simulink model "SplROMInt"  (Simulink 4.00)
settings: Solver=FixedStepDiscrete  StartTime=0.0  StopTime=1024  RelTol=1e-3
libraries: bus_alteradspbuilder x56, store_alteradspbuilder x51, arithm_alteradspbuilder x13
Description:
  | 10 разрядный сплайн-интерполятор
  | Увеличивает частоту дискретизации в кратное двум
  | число раз
  | Использована интерполяция кубическим эрмитовым
  | сплайном
settings Model: Creator="Igor Shelevitsky  sheleviv@mail.ru"  LastModifiedBy=igors

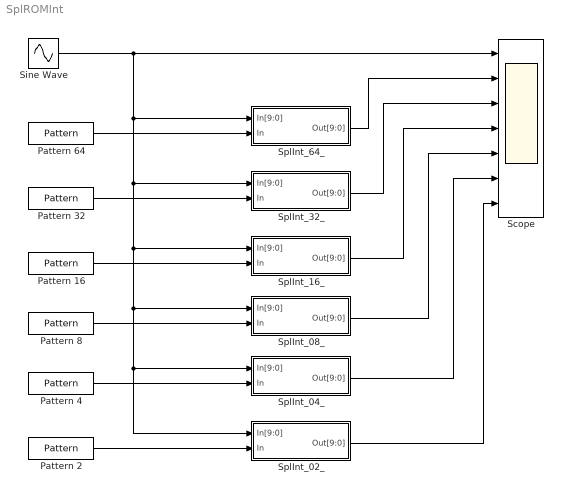
== system SplROMInt ==
  Pattern {2,4,8,16,32,64} (6 alike) : store_alteradspbuilder/Pattern  Priority=28  clken=off  ntsamp=1
  Scope : Scope  NumInputPorts=7
      settings: TimeRange=1024  YMin=-512~-512~-512~-512~-512~-512~-512  YMax=512~512~512~512~512~512~512  SaveToWorkspace=off  SaveName=ScopeData  LimitDataPoints=on  MaxDataPoints=5000
  Sine Wave : Sin  SineType=Time-based  Amplitude=511  Bias=0  Frequency=0.02  Phase=0  Samples=10  SampleTime=1  Offset=0
  SplInt_02_ : Subsystem  AncestorBlock=ALTELINK/AltLab/HDL SubSystem
      settings: RTWFcnNameOpts=Auto  RTWFileNameOpts=Auto
      mask Type: SubSystem AlteraBlockSet
  SplInt_04_ : Subsystem  AncestorBlock=ALTELINK/AltLab/HDL SubSystem
      settings: RTWFcnNameOpts=Auto  RTWFileNameOpts=Auto
      mask Type: SubSystem AlteraBlockSet
  SplInt_08_ : Subsystem  AncestorBlock=ALTELINK/AltLab/HDL SubSystem
      settings: RTWFcnNameOpts=Auto  RTWFileNameOpts=Auto
      mask Type: SubSystem AlteraBlockSet
  SplInt_16_ : Subsystem  AncestorBlock=ALTELINK/AltLab/HDL SubSystem
      settings: RTWFcnNameOpts=Auto  RTWFileNameOpts=Auto
      mask Type: SubSystem AlteraBlockSet
  SplInt_32_ : Subsystem  AncestorBlock=ALTELINK/AltLab/HDL SubSystem
      settings: RTWFcnNameOpts=Auto  RTWFileNameOpts=Auto
      mask Type: SubSystem AlteraBlockSet
  "SplInt_64_ " : Subsystem  AncestorBlock=ALTELINK/AltLab/HDL SubSystem
      settings: RTWFcnNameOpts=Auto  RTWFileNameOpts=Auto
      mask Type: SubSystem AlteraBlockSet
  wires:
  Sine Wave/1 -> "SplInt_64_ "/1(In[9:0]), SplInt_04_/1(In[9:0]), SplInt_02_/1(In[9:0]), SplInt_08_/1(In[9:0]), SplInt_16_/1(In[9:0]), SplInt_32_/1(In[9:0]), Scope/1
  "SplInt_64_ "/1(Out[9:0]) -> Scope/2
  SplInt_32_/1(Out[9:0]) -> Scope/3
  SplInt_16_/1(Out[9:0]) -> Scope/4
  SplInt_08_/1(Out[9:0]) -> Scope/5
  SplInt_04_/1(Out[9:0]) -> Scope/6
  SplInt_02_/1(Out[9:0]) -> Scope/7
  Pattern 64/1 -> "SplInt_64_ "/2(In)
  Pattern 32/1 -> SplInt_32_/2(In)
  Pattern 16/1 -> SplInt_16_/2(In)
  Pattern 8/1 -> SplInt_08_/2(In)
  Pattern 4/1 -> SplInt_04_/2(In)
  Pattern 2/1 -> SplInt_02_/2(In)

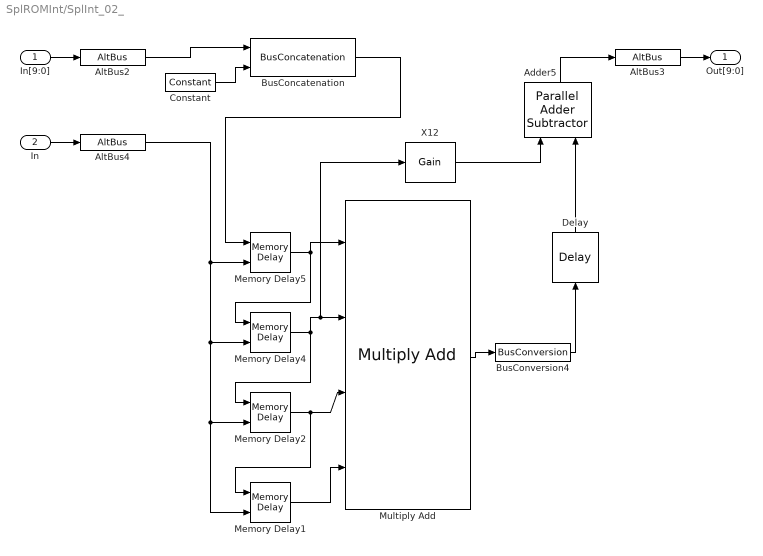
== system SplROMInt/SplInt_02_ ==
  In[9:0] : Inport  Port=1  LatchInput=off
  In : Inport  Port=2  LatchInput=off
  Adder5 : arithm_alteradspbuilder/Parallel  Adder Subtractor  Orientation=up  Inputs=2  direction=++  pipeline=off  clken=off  MaskValue=1
  AltBus2 : bus_alteradspbuilder/AltBus  Description=Sign Binary Fractionnal  sgn=Signed Integer  nodetype=Input Port  bwl=10  bwr=8  sat=off  rnd=off  bp=off  mask_cst=0  LocPin=any  cst=0  modulename=AltBus2  nSgCpl=0
  AltBus3 : bus_alteradspbuilder/AltBus  Description=Sign Binary Fractionnal  sgn=Signed Integer  nodetype=Output Port  bwl=10  bwr=8  sat=off  rnd=off  bp=off  mask_cst=0  LocPin=any  cst=0  modulename=AltBus3  nSgCpl=0
  AltBus4 : bus_alteradspbuilder/AltBus  Description=Sign Binary Fractionnal  sgn=Single Bit  nodetype=Input Port  bwl=1  bwr=0  sat=off  rnd=off  bp=off  mask_cst=0  LocPin=any  cst=0  modulename=AltBus4  nSgCpl=0
  BusConcatenation : bus_alteradspbuilder/BusConcatenation  bwl=10  bwr=4  blean=on
  BusConversion4 : bus_alteradspbuilder/BusConversion  Inputs=Signed Integer  bwl=26  bwr=8  Outputs=Signed Integer  obwl=10  obwr=0  msb=25  lsb=16  rnd=off  sat=off
  Constant : bus_alteradspbuilder/Constant  Description=Sign Binary Fractionnal  sgn=Unsigned Integer  nodetype=Constant  bwl=4  bwr=8  sat=off  rnd=off  bp=off  mask_cst=0  ncstsamp=1  cst=0  modulename=Constant  nSgCpl=0
  Delay : store_alteradspbuilder/Delay  Orientation=up  depth=1  clken=off  MaskValue=1
  Memory Delay{1..2,4..5} (4 alike) : store_alteradspbuilder/Memory Delay  bwaddr=1  depth=1  cst=off  clken=on  eab=on  vDepthAltr=1
  Multiply Add : arithm_alteradspbuilder/Multiply Add  depth=4  BusType=Signed Integer  bwl=14  bwr=0  direction=Add Add  pipeline=No Register  clken=off  eab=off  cst=on  Constantvalues=[-256 2304 2304 -256]  gain=[-256.000000,2304.000000,2304.000000,-256.000000]
  X12 : arithm_alteradspbuilder/Gain  vgain=4096  BusType=Signed Integer  bwl=14  bwr=0  pipeline=0  lpm=off  clken=off  gain=4096  MaskValue=1
  Out[9:0] : Outport  Port=1
  wires:
  AltBus3/1 -> Out[9:0]/1
  In[9:0]/1 -> AltBus2/1
  Multiply Add/1 -> BusConversion4/1
  Memory Delay5/1 -> Memory Delay4/1, Multiply Add/1
  Memory Delay4/1 -> Memory Delay2/1, Multiply Add/2, X12/1
  Memory Delay2/1 -> Memory Delay1/1, Multiply Add/3
  Memory Delay1/1 -> Multiply Add/4
  In/1 -> AltBus4/1
  BusConversion4/1 -> Delay/1
  AltBus4/1 -> Memory Delay5/2, Memory Delay4/2, Memory Delay1/2, Memory Delay2/2
  Constant/1 -> BusConcatenation/2
  AltBus2/1 -> BusConcatenation/1
  BusConcatenation/1 -> Memory Delay5/1
  Adder5/1 -> AltBus3/1
  Delay/1 -> Adder5/2
  X12/1 -> Adder5/1

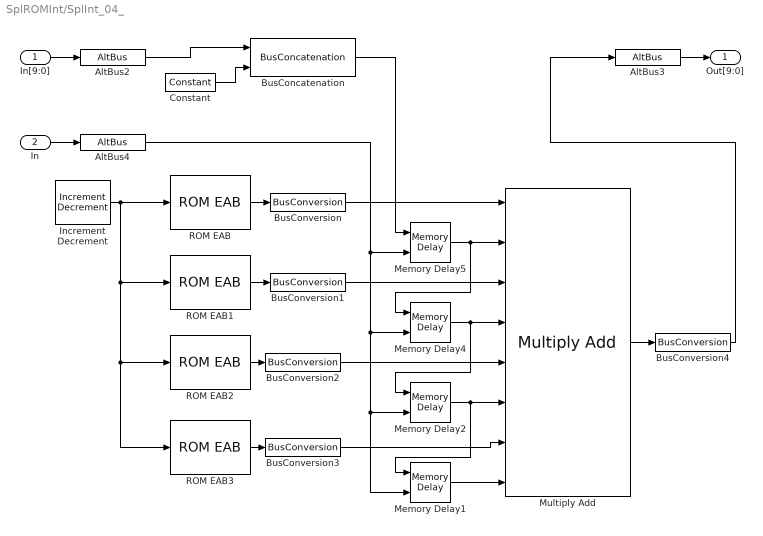
== system SplROMInt/SplInt_04_ ==
  In[9:0] : Inport  Port=1  LatchInput=off
  In : Inport  Port=2  LatchInput=off
  AltBus2 : bus_alteradspbuilder/AltBus  Description=Sign Binary Fractionnal  sgn=Signed Integer  nodetype=Input Port  bwl=10  bwr=8  sat=off  rnd=off  bp=off  mask_cst=0  LocPin=any  cst=0  modulename=AltBus2  nSgCpl=0
  AltBus3 : bus_alteradspbuilder/AltBus  Description=Sign Binary Fractionnal  sgn=Signed Integer  nodetype=Output Port  bwl=10  bwr=8  sat=off  rnd=off  bp=off  mask_cst=0  LocPin=any  cst=0  modulename=AltBus3  nSgCpl=0
  AltBus4 : bus_alteradspbuilder/AltBus  Description=Sign Binary Fractionnal  sgn=Single Bit  nodetype=Input Port  bwl=1  bwr=0  sat=off  rnd=off  bp=off  mask_cst=0  LocPin=any  cst=0  modulename=AltBus4  nSgCpl=0
  BusConcatenation : bus_alteradspbuilder/BusConcatenation  bwl=10  bwr=4  blean=on
  BusConversion{,1..3} (4 alike) : bus_alteradspbuilder/BusConversion  Inputs=Signed Integer  bwl=16  bwr=8  Outputs=Signed Integer  obwl=14  obwr=0  msb=13  lsb=0  rnd=off  sat=off
  BusConversion4 : bus_alteradspbuilder/BusConversion  Inputs=Signed Integer  bwl=26  bwr=8  Outputs=Signed Integer  obwl=10  obwr=0  msb=25  lsb=16  rnd=off  sat=off
  Constant : bus_alteradspbuilder/Constant  Description=Sign Binary Fractionnal  sgn=Unsigned Integer  nodetype=Constant  bwl=4  bwr=8  sat=off  rnd=off  bp=off  mask_cst=0  ncstsamp=1  cst=0  modulename=Constant  nSgCpl=0
  Increment Decrement : arithm_alteradspbuilder/Increment Decrement  BusType=Unsigned Integer  bwl=2  bwr=4  direction=Increment  cst=0  clken=off  ntsamp=1  MaskValue=1
  Memory Delay{1..2,4..5} (4 alike) : store_alteradspbuilder/Memory Delay  bwaddr=1  depth=1  cst=off  clken=on  eab=on  vDepthAltr=1
  Multiply Add : arithm_alteradspbuilder/Multiply Add  depth=4  BusType=Signed Integer  bwl=14  bwr=0  direction=Add Add  pipeline=No Register  clken=off  eab=off  cst=off  Constantvalues=[1 1 1 1]  gain=[1.000000,1.000000,1.000000,1.000000]
  ROM EAB : store_alteradspbuilder/ROM EAB  BusType=Signed Integer  bwl=16  bwr=0  bwaddr=2  Inputs=spl00404.hex  MaskValue=1
  ROM EAB1 : store_alteradspbuilder/ROM EAB  BusType=Signed Integer  bwl=16  bwr=0  bwaddr=2  Inputs=spl00403.hex  MaskValue=1
  ROM EAB2 : store_alteradspbuilder/ROM EAB  BusType=Signed Integer  bwl=16  bwr=0  bwaddr=2  Inputs=spl00402.hex  MaskValue=1
  ROM EAB3 : store_alteradspbuilder/ROM EAB  BusType=Signed Integer  bwl=16  bwr=0  bwaddr=2  Inputs=spl00401.hex  MaskValue=1
  Out[9:0] : Outport  Port=1
  wires:
  AltBus3/1 -> Out[9:0]/1
  In[9:0]/1 -> AltBus2/1
  Increment Decrement/1 -> ROM EAB/1, ROM EAB1/1, ROM EAB2/1, ROM EAB3/1
  ROM EAB/1 -> BusConversion/1
  ROM EAB1/1 -> BusConversion1/1
  ROM EAB2/1 -> BusConversion2/1
  ROM EAB3/1 -> BusConversion3/1
  BusConversion/1 -> Multiply Add/1
  BusConversion1/1 -> Multiply Add/3
  BusConversion2/1 -> Multiply Add/5
  BusConversion3/1 -> Multiply Add/7
  Multiply Add/1 -> BusConversion4/1
  Memory Delay5/1 -> Multiply Add/2, Memory Delay4/1
  Memory Delay4/1 -> Multiply Add/4, Memory Delay2/1
  Memory Delay2/1 -> Multiply Add/6, Memory Delay1/1
  Memory Delay1/1 -> Multiply Add/8
  In/1 -> AltBus4/1
  BusConversion4/1 -> AltBus3/1
  AltBus4/1 -> Memory Delay5/2, Memory Delay4/2, Memory Delay1/2, Memory Delay2/2
  Constant/1 -> BusConcatenation/2
  AltBus2/1 -> BusConcatenation/1
  BusConcatenation/1 -> Memory Delay5/1

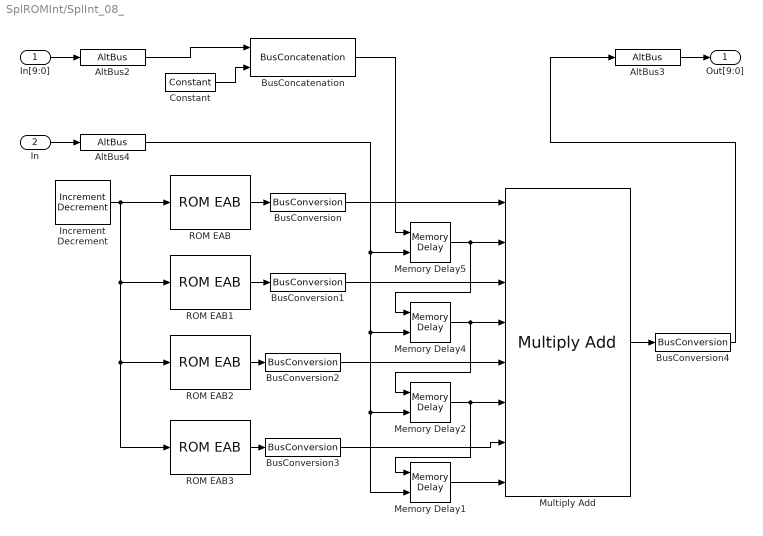
== system SplROMInt/SplInt_08_ ==
  In[9:0] : Inport  Port=1  LatchInput=off
  In : Inport  Port=2  LatchInput=off
  AltBus2 : bus_alteradspbuilder/AltBus  Description=Sign Binary Fractionnal  sgn=Signed Integer  nodetype=Input Port  bwl=10  bwr=8  sat=off  rnd=off  bp=off  mask_cst=0  LocPin=any  cst=0  modulename=AltBus2  nSgCpl=0
  AltBus3 : bus_alteradspbuilder/AltBus  Description=Sign Binary Fractionnal  sgn=Signed Integer  nodetype=Output Port  bwl=10  bwr=8  sat=off  rnd=off  bp=off  mask_cst=0  LocPin=any  cst=0  modulename=AltBus3  nSgCpl=0
  AltBus4 : bus_alteradspbuilder/AltBus  Description=Sign Binary Fractionnal  sgn=Single Bit  nodetype=Input Port  bwl=1  bwr=0  sat=off  rnd=off  bp=off  mask_cst=0  LocPin=any  cst=0  modulename=AltBus4  nSgCpl=0
  BusConcatenation : bus_alteradspbuilder/BusConcatenation  bwl=10  bwr=4  blean=on
  BusConversion{,1..3} (4 alike) : bus_alteradspbuilder/BusConversion  Inputs=Signed Integer  bwl=16  bwr=8  Outputs=Signed Integer  obwl=14  obwr=0  msb=13  lsb=0  rnd=off  sat=off
  BusConversion4 : bus_alteradspbuilder/BusConversion  Inputs=Signed Integer  bwl=26  bwr=8  Outputs=Signed Integer  obwl=10  obwr=0  msb=25  lsb=16  rnd=off  sat=off
  Constant : bus_alteradspbuilder/Constant  Description=Sign Binary Fractionnal  sgn=Unsigned Integer  nodetype=Constant  bwl=4  bwr=8  sat=off  rnd=off  bp=off  mask_cst=0  ncstsamp=1  cst=0  modulename=Constant  nSgCpl=0
  Increment Decrement : arithm_alteradspbuilder/Increment Decrement  BusType=Unsigned Integer  bwl=3  bwr=4  direction=Increment  cst=0  clken=off  ntsamp=1  MaskValue=1
  Memory Delay{1..2,4..5} (4 alike) : store_alteradspbuilder/Memory Delay  bwaddr=1  depth=1  cst=off  clken=on  eab=on  vDepthAltr=1
  Multiply Add : arithm_alteradspbuilder/Multiply Add  depth=4  BusType=Signed Integer  bwl=14  bwr=0  direction=Add Add  pipeline=No Register  clken=off  eab=off  cst=off  Constantvalues=[1 1 1 1]  gain=[1.000000,1.000000,1.000000,1.000000]
  ROM EAB : store_alteradspbuilder/ROM EAB  BusType=Signed Integer  bwl=16  bwr=0  bwaddr=3  Inputs=spl00804.hex  MaskValue=1
  ROM EAB1 : store_alteradspbuilder/ROM EAB  BusType=Signed Integer  bwl=16  bwr=0  bwaddr=3  Inputs=spl00803.hex  MaskValue=1
  ROM EAB2 : store_alteradspbuilder/ROM EAB  BusType=Signed Integer  bwl=16  bwr=0  bwaddr=3  Inputs=spl00802.hex  MaskValue=1
  ROM EAB3 : store_alteradspbuilder/ROM EAB  BusType=Signed Integer  bwl=16  bwr=0  bwaddr=3  Inputs=spl00801.hex  MaskValue=1
  Out[9:0] : Outport  Port=1
  wires:
  AltBus3/1 -> Out[9:0]/1
  In[9:0]/1 -> AltBus2/1
  Increment Decrement/1 -> ROM EAB/1, ROM EAB1/1, ROM EAB2/1, ROM EAB3/1
  ROM EAB/1 -> BusConversion/1
  ROM EAB1/1 -> BusConversion1/1
  ROM EAB2/1 -> BusConversion2/1
  ROM EAB3/1 -> BusConversion3/1
  BusConversion/1 -> Multiply Add/1
  BusConversion1/1 -> Multiply Add/3
  BusConversion2/1 -> Multiply Add/5
  BusConversion3/1 -> Multiply Add/7
  Multiply Add/1 -> BusConversion4/1
  Memory Delay5/1 -> Multiply Add/2, Memory Delay4/1
  Memory Delay4/1 -> Multiply Add/4, Memory Delay2/1
  Memory Delay2/1 -> Multiply Add/6, Memory Delay1/1
  Memory Delay1/1 -> Multiply Add/8
  In/1 -> AltBus4/1
  BusConversion4/1 -> AltBus3/1
  AltBus4/1 -> Memory Delay5/2, Memory Delay4/2, Memory Delay1/2, Memory Delay2/2
  Constant/1 -> BusConcatenation/2
  AltBus2/1 -> BusConcatenation/1
  BusConcatenation/1 -> Memory Delay5/1

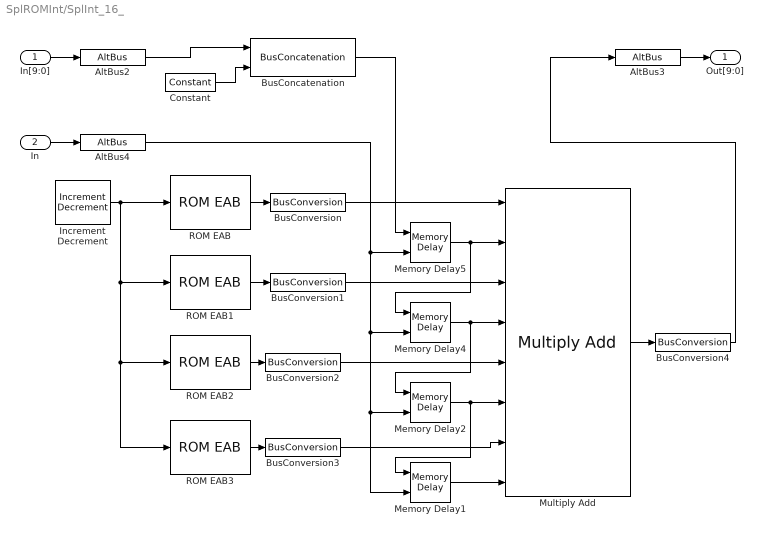
== system SplROMInt/SplInt_16_ ==
  In[9:0] : Inport  Port=1  LatchInput=off
  In : Inport  Port=2  LatchInput=off
  AltBus2 : bus_alteradspbuilder/AltBus  Description=Sign Binary Fractionnal  sgn=Signed Integer  nodetype=Input Port  bwl=10  bwr=8  sat=off  rnd=off  bp=off  mask_cst=0  LocPin=any  cst=0  modulename=AltBus2  nSgCpl=0
  AltBus3 : bus_alteradspbuilder/AltBus  Description=Sign Binary Fractionnal  sgn=Signed Integer  nodetype=Output Port  bwl=10  bwr=8  sat=off  rnd=off  bp=off  mask_cst=0  LocPin=any  cst=0  modulename=AltBus3  nSgCpl=0
  AltBus4 : bus_alteradspbuilder/AltBus  Description=Sign Binary Fractionnal  sgn=Single Bit  nodetype=Input Port  bwl=1  bwr=0  sat=off  rnd=off  bp=off  mask_cst=0  LocPin=any  cst=0  modulename=AltBus4  nSgCpl=0
  BusConcatenation : bus_alteradspbuilder/BusConcatenation  bwl=10  bwr=4  blean=on
  BusConversion{,1..3} (4 alike) : bus_alteradspbuilder/BusConversion  Inputs=Signed Integer  bwl=16  bwr=8  Outputs=Signed Integer  obwl=14  obwr=0  msb=13  lsb=0  rnd=off  sat=off
  BusConversion4 : bus_alteradspbuilder/BusConversion  Inputs=Signed Integer  bwl=26  bwr=8  Outputs=Signed Integer  obwl=10  obwr=0  msb=25  lsb=16  rnd=off  sat=off
  Constant : bus_alteradspbuilder/Constant  Description=Sign Binary Fractionnal  sgn=Unsigned Integer  nodetype=Constant  bwl=4  bwr=8  sat=off  rnd=off  bp=off  mask_cst=0  ncstsamp=1  cst=0  modulename=Constant  nSgCpl=0
  Increment Decrement : arithm_alteradspbuilder/Increment Decrement  BusType=Unsigned Integer  bwl=4  bwr=4  direction=Increment  cst=0  clken=off  ntsamp=1  MaskValue=1
  Memory Delay{1..2,4..5} (4 alike) : store_alteradspbuilder/Memory Delay  bwaddr=1  depth=1  cst=off  clken=on  eab=on  vDepthAltr=1
  Multiply Add : arithm_alteradspbuilder/Multiply Add  depth=4  BusType=Signed Integer  bwl=14  bwr=0  direction=Add Add  pipeline=No Register  clken=off  eab=off  cst=off  Constantvalues=[1 1 1 1]  gain=[1.000000,1.000000,1.000000,1.000000]
  ROM EAB : store_alteradspbuilder/ROM EAB  BusType=Signed Integer  bwl=16  bwr=0  bwaddr=4  Inputs=spl01604.hex  MaskValue=1
  ROM EAB1 : store_alteradspbuilder/ROM EAB  BusType=Signed Integer  bwl=16  bwr=0  bwaddr=4  Inputs=spl01603.hex  MaskValue=1
  ROM EAB2 : store_alteradspbuilder/ROM EAB  BusType=Signed Integer  bwl=16  bwr=0  bwaddr=4  Inputs=spl01602.hex  MaskValue=1
  ROM EAB3 : store_alteradspbuilder/ROM EAB  BusType=Signed Integer  bwl=16  bwr=0  bwaddr=4  Inputs=spl01601.hex  MaskValue=1
  Out[9:0] : Outport  Port=1
  wires:
  AltBus3/1 -> Out[9:0]/1
  In[9:0]/1 -> AltBus2/1
  Increment Decrement/1 -> ROM EAB/1, ROM EAB1/1, ROM EAB2/1, ROM EAB3/1
  ROM EAB/1 -> BusConversion/1
  ROM EAB1/1 -> BusConversion1/1
  ROM EAB2/1 -> BusConversion2/1
  ROM EAB3/1 -> BusConversion3/1
  BusConversion/1 -> Multiply Add/1
  BusConversion1/1 -> Multiply Add/3
  BusConversion2/1 -> Multiply Add/5
  BusConversion3/1 -> Multiply Add/7
  Multiply Add/1 -> BusConversion4/1
  Memory Delay5/1 -> Multiply Add/2, Memory Delay4/1
  Memory Delay4/1 -> Multiply Add/4, Memory Delay2/1
  Memory Delay2/1 -> Multiply Add/6, Memory Delay1/1
  Memory Delay1/1 -> Multiply Add/8
  In/1 -> AltBus4/1
  BusConversion4/1 -> AltBus3/1
  AltBus4/1 -> Memory Delay5/2, Memory Delay4/2, Memory Delay1/2, Memory Delay2/2
  Constant/1 -> BusConcatenation/2
  AltBus2/1 -> BusConcatenation/1
  BusConcatenation/1 -> Memory Delay5/1

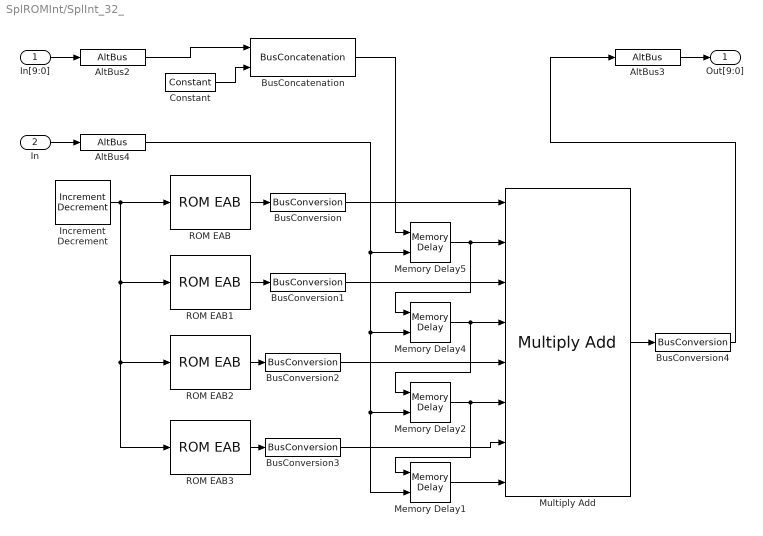
== system SplROMInt/SplInt_32_ ==
  In[9:0] : Inport  Port=1  LatchInput=off
  In : Inport  Port=2  LatchInput=off
  AltBus2 : bus_alteradspbuilder/AltBus  Description=Sign Binary Fractionnal  sgn=Signed Integer  nodetype=Input Port  bwl=10  bwr=8  sat=off  rnd=off  bp=off  mask_cst=0  LocPin=any  cst=0  modulename=AltBus2  nSgCpl=0
  AltBus3 : bus_alteradspbuilder/AltBus  Description=Sign Binary Fractionnal  sgn=Signed Integer  nodetype=Output Port  bwl=10  bwr=8  sat=off  rnd=off  bp=off  mask_cst=0  LocPin=any  cst=0  modulename=AltBus3  nSgCpl=0
  AltBus4 : bus_alteradspbuilder/AltBus  Description=Sign Binary Fractionnal  sgn=Single Bit  nodetype=Input Port  bwl=1  bwr=0  sat=off  rnd=off  bp=off  mask_cst=0  LocPin=any  cst=0  modulename=AltBus4  nSgCpl=0
  BusConcatenation : bus_alteradspbuilder/BusConcatenation  bwl=10  bwr=4  blean=on
  BusConversion{,1..3} (4 alike) : bus_alteradspbuilder/BusConversion  Inputs=Signed Integer  bwl=16  bwr=8  Outputs=Signed Integer  obwl=14  obwr=0  msb=13  lsb=0  rnd=off  sat=off
  BusConversion4 : bus_alteradspbuilder/BusConversion  Inputs=Signed Integer  bwl=26  bwr=8  Outputs=Signed Integer  obwl=10  obwr=0  msb=25  lsb=16  rnd=off  sat=off
  Constant : bus_alteradspbuilder/Constant  Description=Sign Binary Fractionnal  sgn=Unsigned Integer  nodetype=Constant  bwl=4  bwr=8  sat=off  rnd=off  bp=off  mask_cst=0  ncstsamp=1  cst=0  modulename=Constant  nSgCpl=0
  Increment Decrement : arithm_alteradspbuilder/Increment Decrement  BusType=Unsigned Integer  bwl=5  bwr=4  direction=Increment  cst=0  clken=off  ntsamp=1  MaskValue=1
  Memory Delay{1..2,4..5} (4 alike) : store_alteradspbuilder/Memory Delay  bwaddr=1  depth=1  cst=off  clken=on  eab=on  vDepthAltr=1
  Multiply Add : arithm_alteradspbuilder/Multiply Add  depth=4  BusType=Signed Integer  bwl=14  bwr=0  direction=Add Add  pipeline=No Register  clken=off  eab=off  cst=off  Constantvalues=[1 1 1 1]  gain=[1.000000,1.000000,1.000000,1.000000]
  ROM EAB : store_alteradspbuilder/ROM EAB  BusType=Signed Integer  bwl=16  bwr=0  bwaddr=5  Inputs=spl03204.hex  MaskValue=1
  ROM EAB1 : store_alteradspbuilder/ROM EAB  BusType=Signed Integer  bwl=16  bwr=0  bwaddr=5  Inputs=spl03203.hex  MaskValue=1
  ROM EAB2 : store_alteradspbuilder/ROM EAB  BusType=Signed Integer  bwl=16  bwr=0  bwaddr=5  Inputs=spl03202.hex  MaskValue=1
  ROM EAB3 : store_alteradspbuilder/ROM EAB  BusType=Signed Integer  bwl=16  bwr=0  bwaddr=5  Inputs=spl03201.hex  MaskValue=1
  Out[9:0] : Outport  Port=1
  wires:
  AltBus3/1 -> Out[9:0]/1
  In[9:0]/1 -> AltBus2/1
  Increment Decrement/1 -> ROM EAB/1, ROM EAB1/1, ROM EAB2/1, ROM EAB3/1
  ROM EAB/1 -> BusConversion/1
  ROM EAB1/1 -> BusConversion1/1
  ROM EAB2/1 -> BusConversion2/1
  ROM EAB3/1 -> BusConversion3/1
  BusConversion/1 -> Multiply Add/1
  BusConversion1/1 -> Multiply Add/3
  BusConversion2/1 -> Multiply Add/5
  BusConversion3/1 -> Multiply Add/7
  Multiply Add/1 -> BusConversion4/1
  Memory Delay5/1 -> Multiply Add/2, Memory Delay4/1
  Memory Delay4/1 -> Multiply Add/4, Memory Delay2/1
  Memory Delay2/1 -> Multiply Add/6, Memory Delay1/1
  Memory Delay1/1 -> Multiply Add/8
  In/1 -> AltBus4/1
  BusConversion4/1 -> AltBus3/1
  AltBus4/1 -> Memory Delay5/2, Memory Delay4/2, Memory Delay1/2, Memory Delay2/2
  Constant/1 -> BusConcatenation/2
  AltBus2/1 -> BusConcatenation/1
  BusConcatenation/1 -> Memory Delay5/1

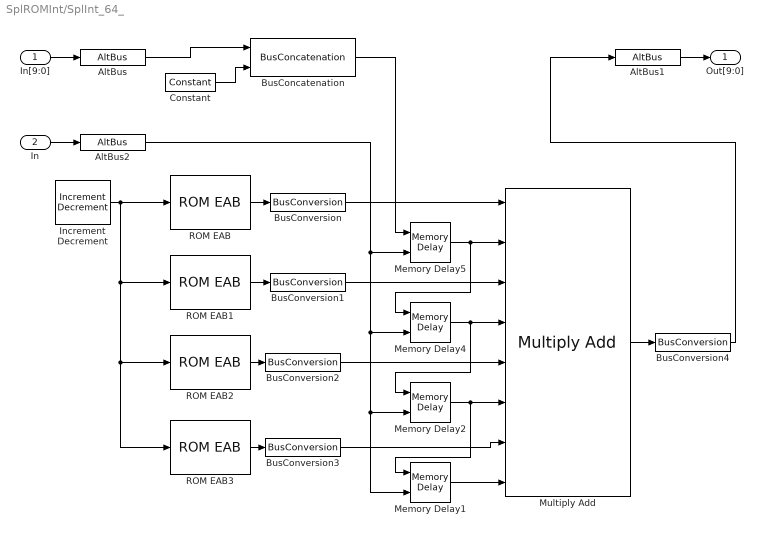
== system SplROMInt/SplInt_64_  ==
  In[9:0] : Inport  Port=1  LatchInput=off
  In : Inport  Port=2  LatchInput=off
  AltBus : bus_alteradspbuilder/AltBus  Description=Sign Binary Fractionnal  sgn=Signed Integer  nodetype=Input Port  bwl=10  bwr=8  sat=off  rnd=off  bp=off  mask_cst=0  LocPin=any  cst=0  modulename=AltBus  nSgCpl=0
  AltBus1 : bus_alteradspbuilder/AltBus  Description=Sign Binary Fractionnal  sgn=Signed Integer  nodetype=Output Port  bwl=10  bwr=8  sat=off  rnd=off  bp=off  mask_cst=0  LocPin=any  cst=0  modulename=AltBus1  nSgCpl=0
  AltBus2 : bus_alteradspbuilder/AltBus  Description=Sign Binary Fractionnal  sgn=Single Bit  nodetype=Input Port  bwl=1  bwr=0  sat=off  rnd=off  bp=off  mask_cst=0  LocPin=any  cst=0  modulename=AltBus2  nSgCpl=0
  BusConcatenation : bus_alteradspbuilder/BusConcatenation  bwl=10  bwr=4  blean=on
  BusConversion{,1..3} (4 alike) : bus_alteradspbuilder/BusConversion  Inputs=Signed Integer  bwl=16  bwr=8  Outputs=Signed Integer  obwl=14  obwr=0  msb=13  lsb=0  rnd=off  sat=off
  BusConversion4 : bus_alteradspbuilder/BusConversion  Inputs=Signed Integer  bwl=26  bwr=8  Outputs=Signed Integer  obwl=10  obwr=0  msb=25  lsb=16  rnd=off  sat=off
  Constant : bus_alteradspbuilder/Constant  Description=Sign Binary Fractionnal  sgn=Unsigned Integer  nodetype=Constant  bwl=4  bwr=8  sat=off  rnd=off  bp=off  mask_cst=0  ncstsamp=1  cst=0  modulename=Constant  nSgCpl=0
  Increment Decrement : arithm_alteradspbuilder/Increment Decrement  BusType=Unsigned Integer  bwl=6  bwr=4  direction=Increment  cst=0  clken=off  ntsamp=1  MaskValue=1
  Memory Delay{1..2,4..5} (4 alike) : store_alteradspbuilder/Memory Delay  bwaddr=1  depth=1  cst=off  clken=on  eab=on  vDepthAltr=1
  Multiply Add : arithm_alteradspbuilder/Multiply Add  depth=4  BusType=Signed Integer  bwl=14  bwr=0  direction=Add Add  pipeline=No Register  clken=off  eab=off  cst=off  Constantvalues=[1 1 1 1]  gain=[1.000000,1.000000,1.000000,1.000000]
  ROM EAB : store_alteradspbuilder/ROM EAB  BusType=Signed Integer  bwl=16  bwr=0  bwaddr=6  Inputs=spl06404.hex  MaskValue=1
  ROM EAB1 : store_alteradspbuilder/ROM EAB  BusType=Signed Integer  bwl=16  bwr=0  bwaddr=6  Inputs=spl06403.hex  MaskValue=1
  ROM EAB2 : store_alteradspbuilder/ROM EAB  BusType=Signed Integer  bwl=16  bwr=0  bwaddr=6  Inputs=spl06402.hex  MaskValue=1
  ROM EAB3 : store_alteradspbuilder/ROM EAB  BusType=Signed Integer  bwl=16  bwr=0  bwaddr=6  Inputs=spl06401.hex  MaskValue=1
  Out[9:0] : Outport  Port=1
  wires:
  AltBus1/1 -> Out[9:0]/1
  In[9:0]/1 -> AltBus/1
  Increment Decrement/1 -> ROM EAB/1, ROM EAB1/1, ROM EAB2/1, ROM EAB3/1
  ROM EAB/1 -> BusConversion/1
  ROM EAB1/1 -> BusConversion1/1
  ROM EAB2/1 -> BusConversion2/1
  ROM EAB3/1 -> BusConversion3/1
  BusConversion/1 -> Multiply Add/1
  BusConversion1/1 -> Multiply Add/3
  BusConversion2/1 -> Multiply Add/5
  BusConversion3/1 -> Multiply Add/7
  Multiply Add/1 -> BusConversion4/1
  Memory Delay5/1 -> Multiply Add/2, Memory Delay4/1
  Memory Delay4/1 -> Multiply Add/4, Memory Delay2/1
  Memory Delay2/1 -> Multiply Add/6, Memory Delay1/1
  Memory Delay1/1 -> Multiply Add/8
  In/1 -> AltBus2/1
  BusConversion4/1 -> AltBus1/1
  AltBus2/1 -> Memory Delay5/2, Memory Delay4/2, Memory Delay1/2, Memory Delay2/2
  Constant/1 -> BusConcatenation/2
  AltBus/1 -> BusConcatenation/1
  BusConcatenation/1 -> Memory Delay5/1
